simulink model "moterhomework"  (R2023b)
settings: Solver=VariableStepAuto  StartTime=0.0  StopTime=10.0  RelTol=1e-3
values from neighbouring files (symbols this model uses):
  b = 0.1    [homeworkone.m]    (also in robotics_0911.m)
  J = 0.2    [homeworkone.m]    (also in robotics_0911.m)
  Ke = 1    [homeworkone.m]    (also in robotics_0911.m)
  Kt = 1    [homeworkone.m]    (also in robotics_0911.m)
  La = 1    [homeworkone.m]    (also in robotics_0911.m)
  Ra = 0.01    [homeworkone.m]    (also in robotics_0911.m)
  Tl = 0    [homeworkone.m]    (also in robotics_0911.m)
  Va = 1    [homeworkone.m]    (also in robotics_0911.m)
settings Model: Creator=junseo  LastModifiedBy=minjs
settings OptimizationCC: ReuseModelBlockBuffer=off

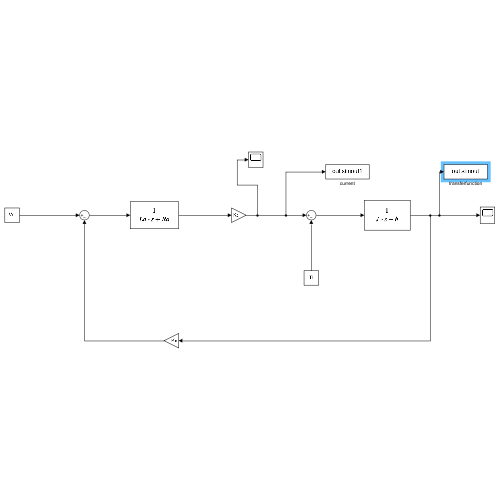
[thumbnail: Simulink's stored preview of the top-level diagram]
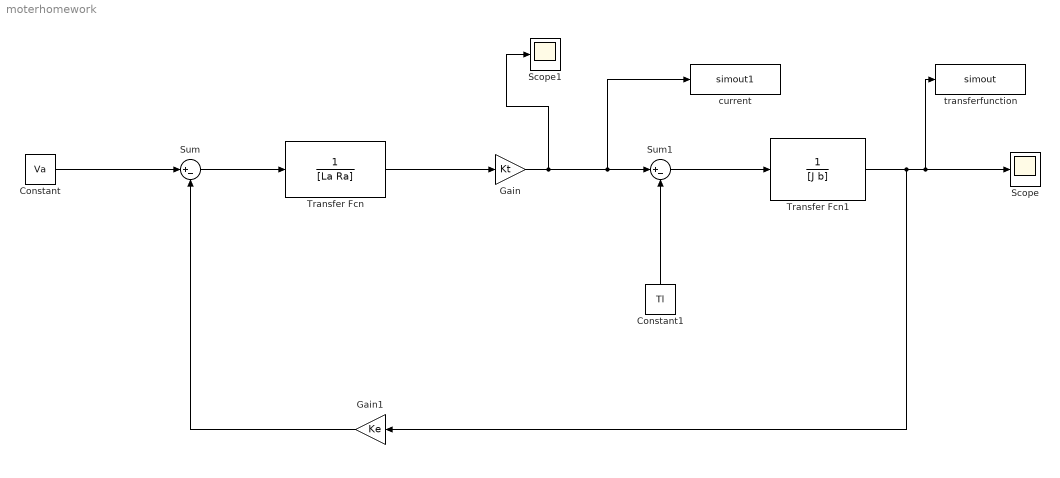
== system moterhomework ==
  Constant : Constant  Value=Va
  Constant1 : Constant  Value=Tl
  Gain : Gain  Gain=Kt
  Gain1 : Gain  Gain=Ke
  Scope : Scope
  Scope1 : Scope
  Sum : Sum  Inputs=|+-
  Sum1 : Sum  Inputs=|+-
  Transfer Fcn : TransferFcn  Denominator=[La Ra]
  Transfer Fcn1 : TransferFcn  Denominator=[J b]
  current : ToWorkspace  VariableName=simout1  SaveFormat=Timeseries  SampleTime=-1
  transferfunction : ToWorkspace  VariableName=simout  SaveFormat=Timeseries  SampleTime=-1
  wires:
  Constant/1 -> Sum/1
  Sum/1 -> Transfer Fcn/1
  Transfer Fcn/1 -> Gain/1
  Gain/1 -> Scope1/1, Sum1/1, current/1
  Sum1/1 -> Transfer Fcn1/1
  Constant1/1 -> Sum1/2
  Transfer Fcn1/1 -> Gain1/1, transferfunction/1, Scope/1
  Gain1/1 -> Sum/2
